simulink model "rslqrModel"  (R2019a)
settings: Solver=ode5  StartTime=0.0  StopTime=10  FixedStep=0.01  RelTol=1e-3
values from neighbouring files (symbols this model uses):
  k_fb = kLqr(:,3:8)    [rslqrScript.m]
  ki_beta = kLqr(:,2)    [rslqrScript.m]
  ki_phi = kLqr(:,1)    [rslqrScript.m]
  sys_actPlusAirframe = series(sys_act,sys_ba)    [rslqrScript.m]
settings Model: Creator=fischer  LastModifiedBy=fischer

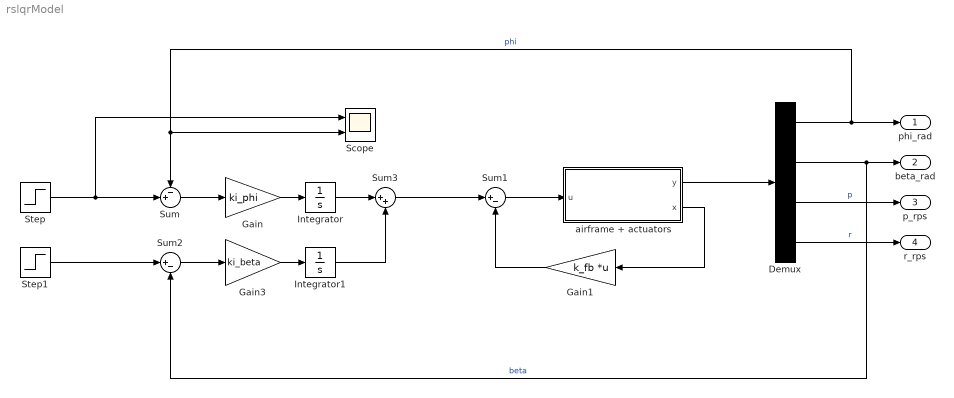
== system rslqrModel ==
  Demux : Demux
  Gain : Gain  Gain=ki_phi
  Gain1 : Gain  Gain=k_fb  Multiplication=Matrix(K*u)
  Gain3 : Gain  Gain=ki_beta
  Integrator : Integrator
  Integrator1 : Integrator
  Scope : Scope  NumInputPorts=2
  Step : Step  Time=2  SampleTime=0
  Step1 : Step  After=0  SampleTime=0
  Sum : Sum  Inputs=-+|
  Sum1 : Sum  Inputs=|+-
  Sum2 : Sum  Inputs=|+-
  Sum3 : Sum  Inputs=|++
  airframe + actuators : Subsystem  mask{A=sys_actPlusAirframe.A, B=sys_actPlusAirframe.B, C=sys_actPlusAirframe.C, D=sys_actPlusAirframe.D}
      mask Display:
      | disp('xDot = Ax + Bu\n\n');
      | 
      | disp('y = Cx + Du');
  phi_rad : Outport
  beta_rad : Outport  Port=2
  p_rps : Outport  Port=3
  r_rps : Outport  Port=4
  wires:
  Integrator/1 -> Sum3/1
  airframe + actuators/1(y) -> Demux/1
  Sum1/1 -> airframe + actuators/1(u)
  Demux/1 -> phi_rad/1, Scope/2, Sum/1  "phi"
  Demux/3 -> p_rps/1  "p"
  Sum/1 -> Gain/1
  Gain/1 -> Integrator/1
  Gain1/1 -> Sum1/2
  airframe + actuators/2(x) -> Gain1/1
  Sum2/1 -> Gain3/1
  Gain3/1 -> Integrator1/1
  Integrator1/1 -> Sum3/2
  Sum3/1 -> Sum1/1
  Demux/2 -> beta_rad/1, Sum2/2  "beta"
  Demux/4 -> r_rps/1  "r"
  Step/1 -> Scope/1, Sum/2
  Step1/1 -> Sum2/1

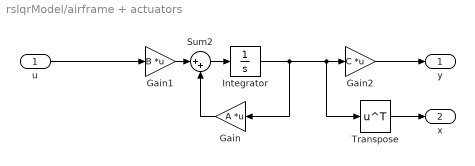
== system rslqrModel/airframe + actuators ==
  u : Inport
  Gain : Gain  Gain=A  Multiplication=Matrix(K*u)
  Gain1 : Gain  Gain=B  Multiplication=Matrix(K*u)
  Gain2 : Gain  Gain=C  Multiplication=Matrix(K*u)
  Integrator : Integrator
  Sum2 : Sum  Inputs=|++
  Transpose : Math  Operator=transpose  SaturateOnIntegerOverflow=on
  y : Outport
  x : Outport  Port=2
  wires:
  Sum2/1 -> Integrator/1
  Gain1/1 -> Sum2/1
  Integrator/1 -> Gain/1, Transpose/1, Gain2/1
  Gain/1 -> Sum2/2
  Gain2/1 -> y/1
  u/1 -> Gain1/1
  Transpose/1 -> x/1
